simulink model "RocketSim2"  (R2020b)
settings: Solver=VariableStepAuto  StartTime=0.0  StopTime=10.0  RelTol=1e-3
libraries: simulink x2, simulink_extras x2, shared3dof x1
settings Model: Creator=bowen  LastModifiedBy=bowen

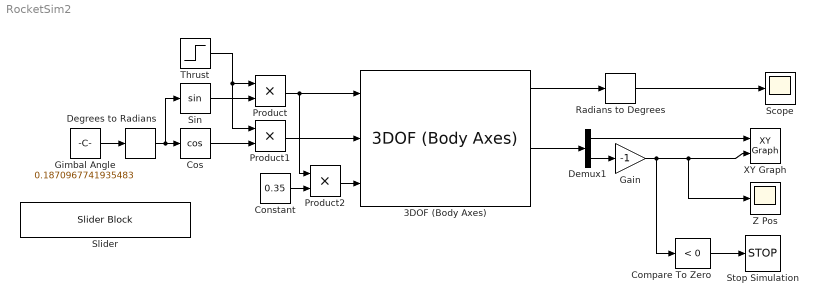
== system RocketSim2 ==
  3DOF (Body Axes) : shared3dof/3DOF (Body Axes)  units=Metric (MKS)  mtype=Fixed  v_ini=0  theta_ini=0  alpha_ini=0  pos_ini=[0 0]  q_ini=0  mass=0.7  mass_e=0.5  mass_f=3.0  Iyy=0.113  Iyy_e=0.5  Iyy_f=3.0  g_in=Internal  g=9.81  vre_flag=on  abi_flag=off  aMode=0  vel_statename=''  theta_statename=''  pos_statename=''  q_statename=''  mass_statename=''
      settings: SourceProductBaseCode=AE,PW,MT,UV,VE,VP
  Compare To Zero : simulink/Logic and Bit Operations/Compare To Zero  relop=<  OutDataTypeStr=boolean
  Constant : Constant  Value=0.35
  Cos : Trigonometry  Operator=cos
  Degrees to Radians : simulink_extras/Transformations/Degrees to Radians
  Demux1 : Demux  Outputs=2
  Gain : Gain  Gain=-1
  Gimbal Angle : Constant  Value=0.1870967741935483
  Product : Product
  Product1 : Product
  Product2 : Product
  Radians to Degrees : simulink_extras/Transformations/Radians to Degrees
  Scope : Scope
  Sin : Trigonometry
  Slider : SliderBlock  ScaleMin=-1  ScaleMax=1
  Stop Simulation : Stop
  Thrust : Step  Time=2  Before=-15  After=0  SampleTime=0
  XY Graph : simulink/Sinks/XY Graph  xmin=-50  xmax=50  ymin=0  ymax=100  st=-1
  Z Pos : Scope
  wires:
  Demux1/2 -> Gain/1
  Gain/1 -> XY Graph/2, Z Pos/1, Compare To Zero/1
  Compare To Zero/1 -> Stop Simulation/1
  Demux1/1 -> XY Graph/1
  3DOF (Body Axes)/4 -> Demux1/1
  Gimbal Angle/1 -> Degrees to Radians/1
  Degrees to Radians/1 -> Sin/1, Cos/1
  Cos/1 -> Product1/2
  Sin/1 -> Product/2
  Product1/1 -> 3DOF (Body Axes)/2
  Product/1 -> Product2/1, 3DOF (Body Axes)/1
  Thrust/1 -> Product1/1, Product/1
  Product2/1 -> 3DOF (Body Axes)/3
  3DOF (Body Axes)/1 -> Radians to Degrees/1
  Radians to Degrees/1 -> Scope/1
  Constant/1 -> Product2/2
